simulink model "ClosedUniverse"  (Simulink 3.00)
settings: Solver=ode45  StartTime=0.0  StopTime=10.0  FixedStep=0.1  MaxStep=0.02  RelTol=1e-3
settings Model: BooleanDataType=on  RTWOptions="-aEnforceIntegerDowncast=1 -aFoldNonRolledExpr=1 -aInlineInvariantSignals=1 -aInlineParameters=0 -aLocalBlockOutputs=1 -aRollThreshold=5 -aZeroInternalMemoryAtStartup=1 -aZeroExternalMemoryAtStartup=1 -aInitFltsAndDblsToZero=1 -aGenerateReport=0 -aGenCodeOnly=0 -aRTWVerbose=1 -aIncludeHyperlinkInReport=0 -aLaunchReport=0 -aForceParamTrailComments=0 -aGenerateComments=1 -aIgnoreCustomStorageClasses=1 -aIncHierarchyInIds=0 -aMaxRTWIdLen=31 -aShowEliminatedStatements=0 -aPrefixModelToSubsysFcnNames=1 -aIncDataTypeInIds=0 -aInsertBlockDesc=0 -aSimulinkBlockComments=1 -aInlinedPrmAccess=\"Literals\"  -aSuppressErrorStatus=0 -aModelReferenceCompliant=1 -aSupportNonInlinedSFcns=1 -aSupportContinuousTime=1 -aSupportComplex=1 -aSupportNonFinite=1 -aSupportAbsoluteTime=1 -aTargetFcnLib=\"ansi_tfl_tmw.mat\" -aMultiInstanceERTCode=0 -aLogVarNameModifier=\"rt_\" -aIsPILTarget=0 -aCombineOutputUpdateFcns=0 -aGenerateASAP2=0 -aGenerateSampleERTMain=0 -aGenerateFullHeader=1 -aUtilityFuncGeneration=\"Auto\" -aIncludeFileDelimiter=\"Auto\" -aIncludeMdlTerminateFcn=1 -aPurelyIntegerCode=0 -aERTCustomFileBanners=0 -aRTWCAPIStates=0 -aRTWCAPIParams=0 -aRTWCAPISignals=0 -aMatFileLogging=1 -aGenFloatMathFcnCalls=\"ANSI_C\" -aExtModeMexFile=\"ext_comm\" -aExtModeTransport=0 -aExtModeStaticAllocSize=1000000 -aExtModeTesting=0 -aExtModeStaticAlloc=0 -aExtMode=0"  ExtModeTrigMode=normal  ExtModeArmWhenConnect=on  LastModifiedBy=campa

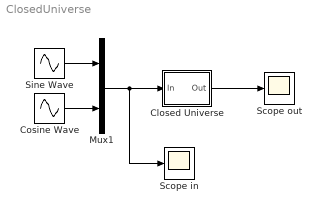
== system ClosedUniverse ==
  Closed Universe : Subsystem  mask(Closed Universe){xmin=[-15 -5], xmax=[15   10]}
      mask prompts: xmin "Min"; xmax "Max"
      mask help:
      | This block wraps the input vector to a given hypercuboid.
      |    When the input is inside the n-dimensional slot defined by the two
      |    limiting vectors Min and Max, then the output is equal to the input.
      |    When the input exceeds a limit along one dimension, the output
      |    reappears "on the other side" of the slot, along the same dimension.
      mask Help:
      | This block wraps the input vector to a given hypercuboid.
      |    When the input is inside the n-dimensional slot defined by the two
      |    limiting vectors Min and Max, then the output is equal to the input.
      |    When the input exceeds a limit along one dimension, the output
      |    reappears "on the other side" of the slot, along the same dimension.
      |    <br><br>
      |    This block is especially useful if you want to limit the evolution of a given
      |    variable in a certain range, for example, when displaying images with the
      |    virtual reality toolbox, it is better to keep the object positions within certain
      |    limits, otherwise numerical problems may prevent a correct visualization.
  Cosine Wave : Sin  Amplitude=10  Frequency=1  Phase=pi/2  SampleTime=0.02
  Mux1 : Mux  Inputs=2
  Scope in : Scope
      settings: TimeRange=10  YMin=-20  YMax=20  SaveToWorkspace=off
  Scope out : Scope
      settings: TimeRange=10  YMin=-15  YMax=15  SaveToWorkspace=off  SaveName=ScopeData
  Sine Wave : Sin  Amplitude=20  Frequency=1  Phase=0  SampleTime=0.02
  wires:
  Sine Wave/1 -> Mux1/1
  Cosine Wave/1 -> Mux1/2
  Mux1/1 -> Scope in/1, Closed Universe/1(In)
  Closed Universe/1(Out) -> Scope out/1

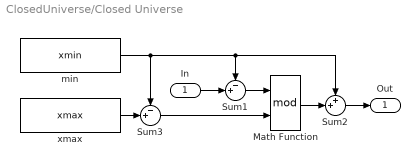
== system ClosedUniverse/Closed Universe ==
  In : Inport  Port=1  PortWidth=-1  SampleTime=-1  DataType=auto
      settings: SignalType=auto
  Math Function : Math  Operator=mod  OutputSignalType=auto
  Sum1 : Sum  Inputs=-+|  SaturateOnIntegerOverflow=on
  Sum2 : Sum  Inputs=++|  SaturateOnIntegerOverflow=on
  Sum3 : Sum  Inputs=-+|  SaturateOnIntegerOverflow=on
  min : Constant  Value=xmin
  xmax : Constant  Value=xmax
  Out : Outport  Port=1
  wires:
  Sum1/1 -> Math Function/1
  min/1 -> Sum3/1, Sum1/1, Sum2/1
  In/1 -> Sum1/2
  xmax/1 -> Sum3/2
  Sum3/1 -> Math Function/2
  Math Function/1 -> Sum2/2
  Sum2/1 -> Out/1
